simulink model "Low_Pass_Filter_Study"  (R2017b)
settings: Solver=VariableStepAuto  StartTime=0.0  StopTime=10.0  RelTol=1e-3
libraries: simulink x2, dsparch4 x1, dspfdesign x1, cstblocks x1
settings Model: Creator=cspt  LastModifiedBy=cspt

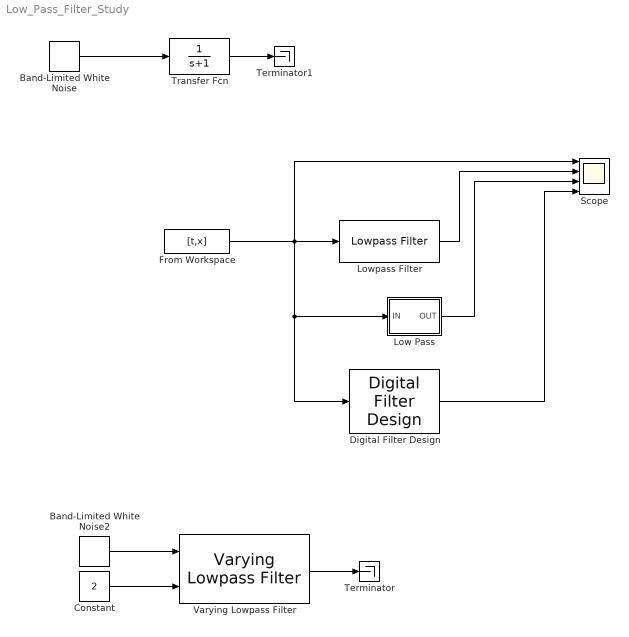
== system Low_Pass_Filter_Study ==
  Band-Limited White Noise : simulink/Sources/Band-Limited White Noise  Cov=[0.1]  Ts=0.1  seed=[23341]
  Band-Limited White Noise2 : simulink/Sources/Band-Limited White Noise  Cov=[0.1]  Ts=0.1  seed=[23341]
  Constant : Constant  Value=2
  Digital Filter Design : dsparch4/Digital Filter Design  mwdsp_browser_bugfix_var=off
  From Workspace : FromWorkspace  VariableName=[t,x]  SampleTime=0.001  Interpolate=off  OutputAfterFinalValue=Setting to zero
  Low Pass : Subsystem  TreatAsAtomicUnit=on
  Lowpass Filter : dspfdesign/Lowpass Filter  FilterType=IIR  DesignForMinimumOrder=off  FilterOrder=3  PassbandFrequency=10  StopbandFrequency=400  PassbandRipple=0.1  StopbandAttenuation=80  InheritSampleRate=on  SampleRate=44100  SimulateUsing=Interpreted execution  roundingMode=Floor  coeffsDataTypeStr=fixdt(1,16)
  Scope : Scope  NumInputPorts=4
  Terminator : Terminator
  Terminator1 : Terminator
  Transfer Fcn : TransferFcn  Denominator=[1 1]
  Varying Lowpass Filter : cstblocks/Linear Parameter Varying/Varying Lowpass Filter  N=1
      settings: SourceProductName=Control System Toolbox
  wires:
  Band-Limited White Noise/1 -> Transfer Fcn/1
  Lowpass Filter/1 -> Scope/2
  Band-Limited White Noise2/1 -> Varying Lowpass Filter/1
  Constant/1 -> Varying Lowpass Filter/2
  From Workspace/1 -> Digital Filter Design/1, Low Pass/1(IN), Scope/1, Lowpass Filter/1
  Varying Lowpass Filter/1 -> Terminator/1
  Transfer Fcn/1 -> Terminator1/1
  Low Pass/1(OUT) -> Scope/3
  Digital Filter Design/1 -> Scope/4

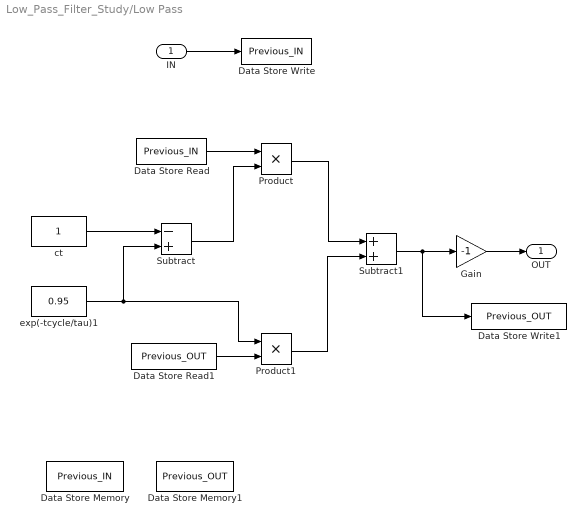
== system Low_Pass_Filter_Study/Low Pass ==
  IN : Inport
  Data Store Memory : DataStoreMemory  DataStoreName=Previous_IN  ReadBeforeWriteMsg=warning  WriteAfterWriteMsg=warning  WriteAfterReadMsg=warning  ShowAdditionalParam=off
  Data Store Memory1 : DataStoreMemory  DataStoreName=Previous_OUT  ReadBeforeWriteMsg=warning  WriteAfterWriteMsg=warning  WriteAfterReadMsg=warning  ShowAdditionalParam=off
  Data Store Read : DataStoreRead  DataStoreName=Previous_IN
  Data Store Read1 : DataStoreRead  DataStoreName=Previous_OUT
  Data Store Write : DataStoreWrite  DataStoreName=Previous_IN
  Data Store Write1 : DataStoreWrite  DataStoreName=Previous_OUT
  Gain : Gain  Gain=-1
  Product : Product
  Product1 : Product
  Subtract : Sum  Inputs=-+
  Subtract1 : Sum
  ct : Constant
  exp(-tcycle/tau)1 : Constant  Value=0.95
  OUT : Outport
  wires:
  IN/1 -> Data Store Write/1
  Data Store Read/1 -> Product/1
  Data Store Read1/1 -> Product1/2
  ct/1 -> Subtract/1
  Subtract/1 -> Product/2
  exp(-tcycle/tau)1/1 -> Product1/1, Subtract/2
  Product/1 -> Subtract1/1
  Product1/1 -> Subtract1/2
  Subtract1/1 -> Gain/1, Data Store Write1/1
  Gain/1 -> OUT/1
